simulink model "mpc_model_with_pos_est"  (R2019a)
settings: Solver=FixedStepAuto  StartTime=0.0  StopTime=Tfinal  RelTol=1e-3
values from neighbouring files (symbols this model uses):
  A = [-0.0285 -0.0014; -0.0371 -0.1476]    [model.m]
  DCLINK_Cap = 1000e-12    (= 1e-09)    [mpc_model_parameters.m]    (also in mpc_model_parameters_dual_module.m = 0.001)
  FaultTime = 50    [mpc_model_parameters.m]
  FluxPM = MeanInducedVoltagePeak/(2*pi*100)    [mpc_model_parameters.m]    (also in mpc_model_parameters_dual_module.m)
  Inertia = 1e-2    (= 0.01)    [mpc_model_parameters.m]    (also in mpc_model_parameters_dual_module.m)
  iqrated = Trated/(1.5*PolePairs*FluxPM)    [mpc_model_parameters.m]    (also in mpc_model_parameters_dual_module.m)
  MeanLq = (1/12)*(Module1Phase_A_Lq+Module1Phase_B_Lq+Module1Phase_C_Lq+     Module2Phase_A_Lq+Module2Phase_B_Lq+Module2Phase_C_Lq+     Module3Phase_A_Lq+Module3Phase_B_Lq+Module3Phase_C_Lq+     Module4Phase_A_Lq+Module4Phase_B_Lq+Module4Phase_C_Lq)    [mpc_model_parameters.m]    (also in mpc_model_parameters_dual_module.m)
  PolePairs = 10    [mpc_model_parameters.m]    (also in mpc_model_parameters_dual_module.m)
  Rin = 1e-3    (= 0.001)    [mpc_model_parameters.m]    (also in mpc_model_parameters_dual_module.m)
  Rs = 0.531    [Loss_Distribution.m]    (also in MPC_id_iq.m; mpc_model_parameters.m = 0.321; mpc_model_parameters_dual_module.m = 0.539)
  Sampling_time = 1e-6    (= 1e-06)    [mpc_model_parameters.m]    (also in mpc_model_parameters_dual_module.m)
  SpeedRef1 = 50    [mpc_model_parameters.m]    (also in mpc_model_parameters_dual_module.m = 35)
  SpeedRef2 = 100    [mpc_model_parameters.m]    (also in mpc_model_parameters_dual_module.m = 35)
  SpeedRefUpdateTime = 0.25    [mpc_model_parameters.m]    (also in mpc_model_parameters_dual_module.m = 1.75)
  Tload1 = 5    [mpc_model_parameters.m]    (also in mpc_model_parameters_dual_module.m = 30)
  Tload2 = 10    [mpc_model_parameters.m]    (also in mpc_model_parameters_dual_module.m = 63.6619772368)
  TloadUpdateTime = 0.5    [mpc_model_parameters.m]    (also in mpc_model_parameters_dual_module.m)
  Vdc = 50    [mpc_model_parameters.m]    (also in mpc_model_parameters_dual_module.m = 40)
  Vin = Vdc + Rin*(Pout/Vdc)    (= 50.04)    [mpc_model_parameters.m]    (also in mpc_model_parameters_dual_module.m = 40.05)
  ViscousFriction = 1e-3    (= 0.001)    [mpc_model_parameters.m]    (also in mpc_model_parameters_dual_module.m)
undefined symbols (not defined in the file or in its folder): DiscIntNeverNeededParam
libraries: powerlib x16, dspswit3 x6, simulink x2, powerlib_meascontrol x2
settings Model: Creator=hakan  LastModifiedBy=hakan
settings SolverCC: ZeroCrossAlgorithm=Adaptive
settings DebuggingCC: IgnoredZcDiagnostic=none

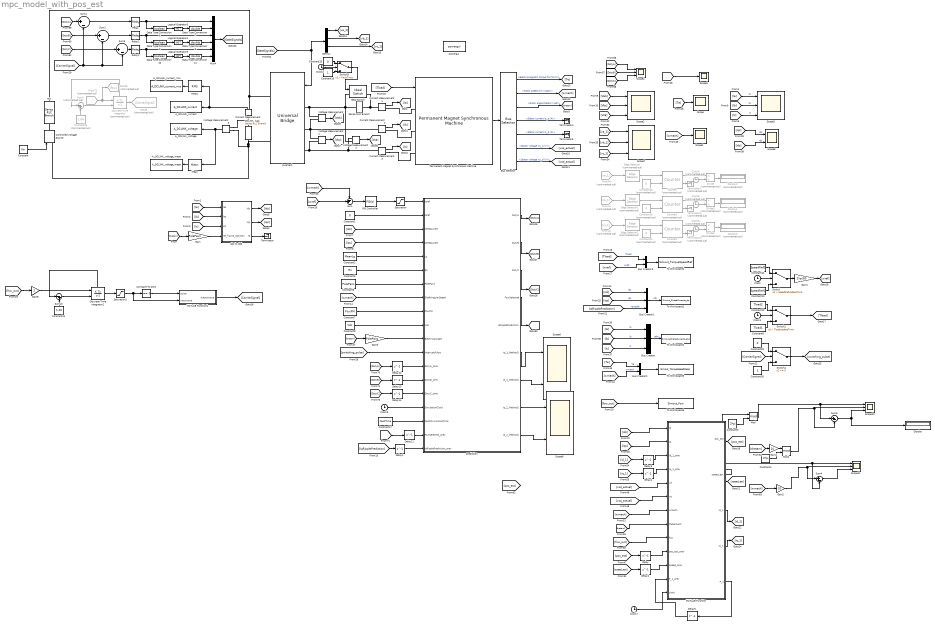
== system mpc_model_with_pos_est ==
  A_DCLINK_current : ToWorkspace  VariableName=A_DCLINK_current  SaveFormat=Structure With Time  SampleTime=-1
  A_DCLINK_current_rms : ToWorkspace  VariableName=A_DCLINK_current_rms  SaveFormat=Structure With Time  SampleTime=-1
  A_DCLINK_voltage : ToWorkspace  VariableName=A_DCLINK_voltage  SaveFormat=Structure With Time  SampleTime=-1
  A_DCLINK_voltage_mean : ToWorkspace  VariableName=A_DCLINK_voltage_mean  SaveFormat=Structure With Time  SampleTime=-1
  Bus Creator : BusCreator  Inputs=3
  Bus Creator1 : BusCreator  Inputs=3
  Bus Creator2 : BusCreator  Inputs=2
  Bus Creator3 : BusCreator  Inputs=2
  Bus Selector : BusSelector  OutputSignals=Electromagnetic torque Te (N*m),Rotor speed wm (rad/s),Rotor angle thetam (rad),Stator current is_q (A),Stator current is_d (A),Stator voltage Vs_q (V),Stator voltage Vs_d (V)
  Clock{,1..3,7} (5 alike) : Clock
  Clock4 : Clock  Commented=on
  Clock5 : Clock  Commented=on
  Clock6 : Clock  Commented=on
  Compare To Zero : simulink/Logic and Bit Operations/Compare To Zero  relop===  OutDataTypeStr=boolean
  Constant : Constant  Value=Vin
  Constant1 : Constant  Value=0
  Constant10 : Constant  Value=SpeedRef1
  Constant11 : Constant  Value=SpeedRef2
  Constant12 : Constant  Value=Tload2
  Constant15 : Constant  Value=0
  Constant16 : Constant
  Constant17 : Constant  Value=FaultTime
  Constant18 : Constant  Commented=on  Value=0
  Constant19 : Constant  Commented=on  Value=0
  Constant2 : Constant  Value=MeanLq
  Constant20 : Constant  Commented=on  Value=0
  Constant24 : Constant  Value=1.02
  Constant26 : Constant  Commented=on  Value=1.04
  Constant29 : Constant  Value=0
  Constant3 : Constant  Value=2*pi
  Constant30 : Constant
  Constant4 : Constant  Value=2*pi
  Constant5 : Constant  Value=Rs
  Constant6 : Constant  Value=PolePairs
  Constant7 : Constant  Value=FluxPM
  Constant8 : Constant  Value=Tload1
  Constant9 : Constant  Value=Vdc
  Controlled Voltage Source : powerlib/Electrical Sources/Controlled Voltage Source  Initialize=on  Source_Type=DC  Amplitude=Vin  Phase=0  Frequency=0  Measurements=None
      settings: SourceProductName=Simscape Electrical
  Counter : dspswit3/Counter  Commented=on  Direction=Up  CountEvent=Rising edge  CounterSize=User defined  MaxCount=9999999999999999999  InitialCount=0  Output=Count and Hit  HitValue=32  ResetInput=on  SamplesPerFrame=1  Ts=1  CntDtype=double  HitDtype=Logical
  Counter1 : dspswit3/Counter  Commented=on  Direction=Up  CountEvent=Rising edge  CounterSize=User defined  MaxCount=9999999999999999999  InitialCount=0  Output=Count and Hit  HitValue=32  ResetInput=on  SamplesPerFrame=1  Ts=1  CntDtype=double  HitDtype=Logical
  Counter2 : dspswit3/Counter  Commented=on  Direction=Up  CountEvent=Rising edge  CounterSize=User defined  MaxCount=9999999999999999999  InitialCount=0  Output=Count and Hit  HitValue=32  ResetInput=on  SamplesPerFrame=1  Ts=1  CntDtype=double  HitDtype=Logical
  Current Measurement{,1..3} (4 alike) : powerlib/Measurements/Current Measurement  PhasorSimulation=off  OutputType=Complex  PSBequivalent=0
      settings: SourceProductName=Simscape Electrical
  DCLINK_Cap : powerlib/Elements/Series RLC Branch  LConnTagsString=__new0  RConnTagsString=__new0  BranchType=C  Resistance=1  Inductance=1e-3  SetiL0=off  InitialCurrent=0  Capacitance=DCLINK_Cap  Setx0=on  InitialVoltage=Vin  Measurements=None
      settings: SourceProductName=Simscape Electrical
  Data Type Conversion10 : DataTypeConversion  OutDataTypeStr=boolean
  Data Type Conversion11 : DataTypeConversion  OutDataTypeStr=double
  Data Type Conversion6 : DataTypeConversion  OutDataTypeStr=boolean
  Data Type Conversion7 : DataTypeConversion  OutDataTypeStr=double
  Data Type Conversion8 : DataTypeConversion  OutDataTypeStr=boolean
  Data Type Conversion9 : DataTypeConversion  OutDataTypeStr=double
  Delay{,1..5,11..14} (10 alike) : Delay  DelayLength=1
  Demux : Demux  Outputs=6
  Discrete-Time Integrator : DiscreteIntegrator  Commented=on  ExternalReset=falling  SampleTime=-1  ShowStatePort=on  ICPrevOutput=DiscIntNeverNeededParam  ICPrevScaledInput=DiscIntNeverNeededParam
  Discrete-Time Integrator2 : DiscreteIntegrator  ExternalReset=falling  SampleTime=Sampling_time  UpperSaturationLimit=1  LowerSaturationLimit=0  ShowStatePort=on  ICPrevOutput=DiscIntNeverNeededParam  ICPrevScaledInput=DiscIntNeverNeededParam
  Display : Display
  Display1 : Display  Commented=on
  Display2 : Display  Commented=on
  Display3 : Display  Commented=on
  Divide : Product  Commented=on  Inputs=*/
  Divide1 : Product  Commented=on  Inputs=*/
  Divide2 : Product  Commented=on  Inputs=*/
  Edge Detector : dspswit3/Edge Detector  Commented=on  InputProcessing=Columns as channels (frame based)
      settings: SourceProductName=DSP System Toolbox  SourceProductBaseCode=DS
  Edge Detector1 : dspswit3/Edge Detector  Commented=on  InputProcessing=Columns as channels (frame based)
      settings: SourceProductName=DSP System Toolbox  SourceProductBaseCode=DS
  Edge Detector2 : dspswit3/Edge Detector  Commented=on  InputProcessing=Columns as channels (frame based)
      settings: SourceProductName=DSP System Toolbox  SourceProductBaseCode=DS
  From40 : From  Commented=on  GotoTag=va_1
  From41 : From  Commented=on  GotoTag=vb_1
  From42 : From  Commented=on  GotoTag=vc_1
  From72 : From  Commented=on  GotoTag=fsw_out
  Gain : Gain  Gain=PolePairs
  Gain1 : Gain  Gain=2*pi/60
  Gain2 : Gain  Gain=10
  Gain3 : Gain  Gain=PolePairs
  Gain4 : Gain  Gain=10
  Gain8 : Gain  Gain=2
  Goto29 : Goto  Commented=on  GotoTag=fsw
  Goto9 : Goto  Commented=on  GotoTag=CarrierSignal
  Ideal Switch : powerlib/Power Electronics/Ideal Switch  Ron=0.001  Lon=0  IC=0  Rs=1e5  Cs=inf  Measurements=on
      settings: SourceProductName=Simscape Electrical
  Inverter1 : powerlib/Power Electronics/Universal Bridge  Arms=3  SnubberResistance=1e5  SnubberCapacitance=inf  Device=IGBT / Diodes  Ron=0.65e-3  Lon=0  ForwardVoltages="[  0  0  ]"  ForwardVoltage=0  GTOparameters=[ 10e-6 , 20e-6 ]  IGBTparameters=[ 1e-6 , 2e-6 ]  Measurements=All voltages and currents  Measurements_2=None  converterType=Rectifier
      settings: SourceProductName=Simscape Electrical
  Logical Operator3 : Logic  Operator=NOT  AllPortsSameDT=off  OutDataTypeStr=boolean
  Logical Operator4 : Logic  Operator=NOT  AllPortsSameDT=off  OutDataTypeStr=boolean
  Logical Operator5 : Logic  Operator=NOT  AllPortsSameDT=off  OutDataTypeStr=boolean
  MATLAB Function : MATLAB Function  TreatAsAtomicUnit=on
  MATLAB Function1 : MATLAB Function  TreatAsAtomicUnit=on
  Mean : powerlib_meascontrol/Measurements/Mean  Freq=THD_mean_frequency  Vinit=0  Ts=0
      settings: SourceProductName=Simscape Electrical
  Mod : Math  Operator=mod  SaturateOnIntegerOverflow=on
  Mod1 : Math  Operator=mod  SaturateOnIntegerOverflow=on
  Mux4 : Mux  Inputs=6
  PID Controller : simulink/Continuous/PID Controller  Controller=PID  Form=Parallel  TimeDomain=Continuous-time  SampleTime=-1  IntegratorMethod=Forward Euler  FilterMethod=Forward Euler  ControllerParametersSource=internal  P=1  I=10  D=0  UseFilter=on  N=100  TunerSelectOption=Transfer Function Based (PID Tuner App)  InitialConditionSource=internal  InitialConditionForIntegrator=0  InitialConditionForFilter=0  DifferentiatorICPrevScaledInput=0  ExternalReset=none  TrackingMode=off  Kt=1  LimitOutput=off  UpperSaturationLimit=inf  LowerSaturationLimit=-inf  LinearizeAsGain=on  AntiWindupMode=none  Kb=1  POutMin=[]  POutMax=[]  IOutMin=[]  IOutMax=[]  DOutMin=[]  DOutMax=[]  NOutMin=[]  NOutMax=[]  SumOutMin=[]  SumOutMax=[]  SaturationOutMin=[]  SaturationOutMax=[]  PParamMin=[]  PParamMax=[]  IParamMin=[]  IParamMax=[]  DParamMin=[]  DParamMax=[]  NParamMin=[]  NParamMax=[]  KbParamMin=[]  KbParamMax=[]  KtParamMin=[]  KtParamMax=[]  KbOutMin=[]  KbOutMax=[]  KtOutMin=[]  KtOutMax=[]  IntegratorOutMin=[]  IntegratorOutMax=[]  FilterOutMin=[]  FilterOutMax=[]  SumI1OutMin=[]  SumI1OutMax=[]  SumI2OutMin=[]  SumI2OutMax=[]  SumI3OutMin=[]  SumI3OutMax=[]  SumI4OutMin=[]  SumI4OutMax=[]  SumDOutMin=[]  SumDOutMax=[]  DifferentiatorOutMin=[]  DifferentiatorOutMax=[]  FilterDiffOutCoefMin=[]  FilterDiffOutCoefMax=[]  ReciprocalOutMin=[]  ReciprocalOutMax=[]  SumDenOutMin=[]  SumDenOutMax=[]  SumNumOutMin=[]  SumNumOutMax=[]  DivideOutMin=[]  DivideOutMax=[]  IntegratorContinuousStateAttributes=''  IntegratorStateMustResolveToSignalObject=off  IntegratorRTWStateStorageClass=Auto  FilterContinuousStateAttributes=''  FilterStateMustResolveToSignalObject=off  FilterRTWStateStorageClass=Auto  ParallelPVariant=InternalParameters  IdealPVariant=Disabled  IVariant=InternalParameters  DVariant=InternalParameters  IntegratorVariant=Continuous  SatVariant=Disabled  AWVariant=Passthrough  PCopyVariant=Disabled  TRVariant=Disabled  FdbkBlocksVariant=Forward  IdealPFdbkVariant=Disabled  SatFdbkVariant=Disabled  DerivativeFilterVariant=ContFilter  NVariant=InternalParameters  NCopyVariant=Disabled  FilterICVariant=InternalICsFilter  IntegratorICVariant=InternalICs  ExternalResetVariant=Disabled  TRSumVariant=Passthrough  SumFdbkVariant=Disabled  SumVariant=Sum_PID
  Permanent Magnet Synchronous Machine : powerlib/Machines/Permanent Magnet Synchronous Machine  NbPhases=3  FluxDistribution=Sinusoidal  RotorType=Round  MechanicalLoad=Torque Tm  PresetModel=No  ShowDetailedParameters=on  MeasurementBus=off  Resistance=Rs  Inductance=8.5e-3  dqInductances=[3.1e-3,3.6e-3]  La=Ls  MachineConstant=Voltage Constant (V_peak L-L / krpm)  Flux=0.18074  VoltageCst=VoltageConstant  TorqueCst=2.7111  Flat=120  Mechanical=[Inertia ViscousFriction PolePairs 0]  PolePairs=4  InitialConditions=[0*100*2*pi/60,0, 0,0]  InitialConditions5ph=[0 0 0 0 0 0]  TsPowergui=0  TsBlock=-1  RefAngle=90 degrees behind phase A axis (modified Park)
  RMS1 : powerlib_meascontrol/Measurements/RMS  TrueRMS=on  Freq=Load_Nominal_Freq  RMSInit=10  Ts=0
      settings: SourceProductName=Simscape Electrical
  Relay : Relay
  Relay1 : Relay
  Relay2 : Relay
  Rin : powerlib/Elements/Series RLC Branch  LConnTagsString=__new0  RConnTagsString=__new0  BranchType=R  Resistance=Rin  Inductance=1e-3  SetiL0=off  InitialCurrent=0  Capacitance=1000e-6  Setx0=off  InitialVoltage=0  Measurements=None
      settings: SourceProductName=Simscape Electrical
  Saturation : Saturate  UpperLimit=2*iqrated  LowerLimit=-2*iqrated  LinearizeAsGain=off
  Saturation1 : Saturate  UpperLimit=1  LowerLimit=0
  Scope : Scope
  Scope1 : Scope
  Scope{2..4,7,10..11} (6 alike) : Scope  NumInputPorts=3
  Scope5 : Scope
  Scope6 : Scope  NumInputPorts=2
  Scope8 : Scope  NumInputPorts=2
  Scope9 : Scope  NumInputPorts=2
  Series RLC Branch : powerlib/Elements/Series RLC Branch  LConnTagsString=__new0  RConnTagsString=__new0  BranchType=R  Resistance=5000  Inductance=1e-3  SetiL0=off  InitialCurrent=0  Capacitance=1e-6  Setx0=off  InitialVoltage=0  Measurements=None
      settings: SourceProductName=Simscape Electrical
  Sum : Sum  Inputs=-+|
  Sum{1..2,4..6} (5 alike) : Sum  Inputs=|+-
  Sum10 : Sum  Inputs=|-+
  Sum3 : Sum  Commented=on  Inputs=|-+
  Switch : Switch  Criteria=u2 > Threshold  Threshold=SpeedRefUpdateTime
  Switch1 : Switch  Criteria=u2 > Threshold  Threshold=TloadUpdateTime
  Switch3 : Switch  Criteria=u2 > Threshold  Threshold=FaultTime
  Switch4 : Switch  Criteria=u2 ~= 0
  Terminator : Terminator
  Terminator1 : Terminator  Commented=on
  Terminator2 : Terminator  Commented=on
  Terminator3 : Terminator  Commented=on
  Terminator4 : Terminator
  Terminator5 : Terminator
  To Workspace1 : ToWorkspace  VariableName=Simout_PhaseCurrents_abc  SaveFormat=Timeseries  SampleTime=-1
  To Workspace2 : ToWorkspace  VariableName=Simout_PhaseCurrents_dq  SaveFormat=Timeseries  SampleTime=-1
  To Workspace3 : ToWorkspace  VariableName=Simout_TorqueSpeedMeas  SaveFormat=Timeseries  SampleTime=-1
  To Workspace4 : ToWorkspace  VariableName=Simout_TorqueSpeedRef  SaveFormat=Timeseries  SampleTime=-1
  To Workspace5 : ToWorkspace  VariableName=Simout_Fsw  SaveFormat=Timeseries  SampleTime=-1
  Voltage Measurement{,1..3} (4 alike) : powerlib/Measurements/Voltage Measurement  PhasorSimulation=off  OutputType=Complex  PSBequivalent=0
      settings: SourceProductName=Simscape Electrical
  abc to dq0 : MATLAB Function  TreatAsAtomicUnit=on
  powergui : powerlib/powergui  Priority=1  SimulationMode=Discrete  SampleTime=Sampling_time  frequency=60  Iterations=50  frequencyindice=0  Pbase=100e6  ErrMax=1e-4  UnitsV=kV  UnitsW=MW  buscounter=0  FunctionMessages=off  echomessages=off  EnableUseOfTLC=off  CurrentSourceSwitches=off  DisableSnubberDevices=off  DisableRonSwitches=off  DisableVfSwitches=off  DisplayEquations=off  AutomaticDiscreteSolvers=off  SolverType=Tustin/Backward Euler (TBE)  Interpol=off  ExternalGateDelay=off  methode=off  Ts=100  x0status=blocks  SPID=on  SwTol=0  HookPort=off  NonlinearTolerance=0  nMaxIteration=15  ContinueOnMaxIteration=off  RestoreLinks=warning  ResistiveCurrentMeasurement=off  Frange=[0:2:500]  Ylog=off  Xlog=on  ShowGrid=off  save=off  variable=ZData  structure=0  ZoomFFT=off  StartTime=0.0  cycles=1  DisplayStyle=1  fundamental=60  FreqAxis=off  MaxFrequency=1000  frequencyindicesteady=1  RmsSteady=1  display=off
      settings: SourceProductName=Simscape Electrical
  prediction : MATLAB Function  TreatAsAtomicUnit=on
  wires:
  Voltage Measurement3/1 -> Mean/1, A_DCLINK_voltage/1
  RMS1/1 -> A_DCLINK_current_rms/1
  Constant/1 -> Controlled Voltage Source/1
  Mean/1 -> A_DCLINK_voltage_mean/1
  Current Measurement/1 -> RMS1/1, A_DCLINK_current/1
  Permanent Magnet Synchronous Machine/1 -> Bus Selector/1
  Bus Selector/1 -> [Te]  "<Electromagnetic torque Te (N*m)>"
  Bus Selector/2 -> [wmech]  "<Rotor speed wm (rad/s)>"
  Current Measurement1/1 -> [Ia]
  Current Measurement2/1 -> [Ib]
  Current Measurement3/1 -> [Ic]
  Bus Selector/3 -> [thetam]  "<Rotor angle thetam (rad)>"
  [thetam] -> Gain/1
  [Ia] -> abc to dq0/1(ias)
  [Ib] -> abc to dq0/2(ibs)
  [Ic] -> abc to dq0/3(ics)
  Gain/1 -> abc to dq0/4(ref_frame_position)
  Bus Selector/4 -> Terminator4/1  "<Stator current is_q (A)>"
  Bus Selector/5 -> Terminator5/1  "<Stator current is_d (A)>"
  abc to dq0/2(iqs) -> [iqs]
  abc to dq0/1(ids) -> [ids]
  abc to dq0/3(i0) -> Terminator/1
  [ids] -> prediction/3(IdMeasured)
  [iqs] -> prediction/4(IqMeasured)
  Constant2/1 -> prediction/5(Ls)
  Voltage Measurement/1 -> [Vab]
  Voltage Measurement1/1 -> [Vbc]
  Voltage Measurement2/1 -> [Vca]
  Bus Selector/6 -> [vsq_actual]  "<Stator voltage Vs_q (V)>"
  Bus Selector/7 -> [vsd_actual]  "<Stator voltage Vs_d (V)>"
  [Vca] -> Scope2/3
  [Vbc] -> Scope2/2
  [Vab] -> Scope2/1
  Constant5/1 -> prediction/6(Rs)
  Constant6/1 -> prediction/7(PolePairs)
  [wmech] -> prediction/8(ShaftAngularSpeed)
  Constant7/1 -> prediction/9(FluxPM)
  Constant9/1 -> prediction/10(Vdc)
  Gain3/1 -> prediction/11(ElectricalAngle)
  [thetam] -> Gain3/1
  [Tload] -> Permanent Magnet Synchronous Machine/1
  PID Controller/1 -> Saturation/1
  Sum/1 -> PID Controller/1
  [wmech] -> Sum/1
  [iqs] -> Bus Creator1/2  "iqs"
  [ids] -> Bus Creator1/1  "ids"
  Constant10/1 -> Switch/3
  Constant11/1 -> Switch/1
  Switch/1 -> Gain1/1
  Clock/1 -> Switch/2
  Clock1/1 -> Switch1/2
  Constant12/1 -> Switch1/1
  Constant8/1 -> Switch1/3
  Switch1/1 -> [Tload]
  Bus Creator/1 -> To Workspace1/1  "Iabc"
  Bus Creator1/1 -> To Workspace2/1  "Idq"
  Bus Creator2/1 -> To Workspace3/1
  [wref] -> Sum/2
  Gain1/1 -> [wref]
  [Tload] -> Bus Creator3/1  "Tload"
  [wref] -> Bus Creator3/2  "wref"
  Bus Creator3/1 -> To Workspace4/1
  [switching_pulse] -> prediction/12(InterruptPulse)
  Clock2/1 -> Switch3/2
  Constant15/1 -> Switch3/1
  Constant16/1 -> Switch3/3
  Switch3/1 -> Ideal Switch/1
  Clock3/1 -> prediction/16(SimulationClock)
  Constant17/1 -> prediction/17(FaultOccuranceTime)
  [va_1] -> Scope7/1
  [vb_1] -> Scope7/2
  [vc_1] -> Scope7/3
  Edge Detector/1 -> Counter/1
  Constant18/1 -> Counter/2
  Counter/1 -> Divide/1
  Clock4/1 -> Divide/2
  Divide/1 -> Display2/1
  [Ib] -> Bus Creator/2  "Ib"
  [Ia] -> Bus Creator/1  "Ia"
  [Ic] -> Bus Creator/3  "Ic"
  [Ib] -> Scope3/2  "Ib"
  [Ic] -> Scope3/3  "Ic"
  [Ia] -> Scope3/1  "Ia"
  [iqs] -> Scope8/1  "iqs"
  [ids] -> Scope8/2  "ids"
  Counter/2 -> Terminator1/1
  From40/1 -> Edge Detector/1
  From41/1 -> Edge Detector1/1
  Counter1/2 -> Terminator2/1
  Divide1/1 -> Display1/1
  Clock5/1 -> Divide1/2
  Counter1/1 -> Divide1/1
  Constant19/1 -> Counter1/2
  Edge Detector1/1 -> Counter1/1
  Edge Detector2/1 -> Counter2/1
  Constant20/1 -> Counter2/2
  Counter2/1 -> Divide2/1
  Clock6/1 -> Divide2/2
  Divide2/1 -> Display3/1
  Counter2/2 -> Terminator3/1
  From42/1 -> Edge Detector2/1
  [Te] -> Bus Creator2/1  "Te"
  [wmech] -> Bus Creator2/2  "wmech"
  [Te] -> Scope/1
  [wmech] -> Scope1/1
  prediction/1(DutyA) -> [DutyA]
  prediction/3(DutyC) -> [DutyC]
  prediction/2(DutyB) -> [DutyB]
  [DutyB] -> Scope4/2
  [DutyA] -> Scope4/1
  [DutyC] -> Scope4/3
  Constant26/1 -> Sum3/2
  From72/1 -> Goto29/1, Discrete-Time Integrator/1
  Discrete-Time Integrator/State -> Sum3/1
  Sum3/1 -> Discrete-Time Integrator/2
  Switch4/1 -> [switching_pulse]
  Constant30/1 -> Switch4/3
  Constant29/1 -> Switch4/1
  [GateSignals] -> Inverter1/1, Demux/1
  Demux/1 -> [va_1]
  Demux/3 -> [vb_1]
  prediction/4(FswSelected) -> [fsw_out]
  Delay11/1 -> prediction/18(FswSelected_prev)
  [fsw_out] -> Delay11/1
  [DutyB] -> Delay13/1
  [DutyA] -> Delay12/1
  [DutyC] -> Delay14/1
  Delay13/1 -> prediction/14(DutyB_prev)
  Delay12/1 -> prediction/13(DutyA_prev)
  Delay14/1 -> prediction/15(DutyC_prev)
  Discrete-Time Integrator/1 -> Goto9/1
  [CarrierSignal] -> Switch4/2
  Demux/5 -> [vc_1]
  [IqRipplePrediction] -> Delay1/1
  Delay1/1 -> prediction/19(IqRipplePrediction_prev)
  [CarrierSignal] -> Sum1/2, Sum2/2, Sum5/2
  Logical Operator4/1 -> Data Type Conversion9/1
  [DutyA] -> Sum1/1
  Data Type Conversion8/1 -> Logical Operator4/1
  Data Type Conversion10/1 -> Logical Operator5/1
  Relay1/1 -> Data Type Conversion8/1, Mux4/3
  Relay2/1 -> Data Type Conversion10/1, Mux4/5
  Data Type Conversion6/1 -> Logical Operator3/1
  Sum1/1 -> Relay/1
  Data Type Conversion11/1 -> Mux4/6
  [DutyC] -> Sum5/1
  Relay/1 -> Mux4/1, Data Type Conversion6/1
  Data Type Conversion9/1 -> Mux4/4
  Sum5/1 -> Relay2/1
  Logical Operator3/1 -> Data Type Conversion7/1
  Logical Operator5/1 -> Data Type Conversion11/1
  Sum2/1 -> Relay1/1
  Mux4/1 -> [GateSignals]
  [DutyB] -> Sum2/1
  Data Type Conversion7/1 -> Mux4/2
  [fsw_out] -> Scope5/1
  Saturation/1 -> prediction/1(iqref)
  Discrete-Time Integrator2/State -> Sum10/1
  Gain8/1 -> Discrete-Time Integrator2/1
  Sum10/1 -> Discrete-Time Integrator2/2
  [fsw_out] -> Gain8/1
  Saturation1/1 -> MATLAB Function1/2(inputwave), Compare To Zero/1
  Constant24/1 -> Sum10/2
  Discrete-Time Integrator2/1 -> Saturation1/1
  Compare To Zero/1 -> MATLAB Function1/1(pulse)
  MATLAB Function1/1(outputwave) -> [CarrierSignal]
  [fsw_out] -> To Workspace5/1
  [IqRipplePrediction] -> Bus Creator1/3  "iqripple"
  Constant1/1 -> prediction/2(idref)
  prediction/7(Id_1_Method1) -> Scope6/2
  prediction/6(Iq_1_Method1) -> Scope6/1
  prediction/8(Iq_2_Method1) -> Scope9/1
  prediction/9(Id_2_Method1) -> Scope9/2
  [ids] -> MATLAB Function/1(id)
  [iqs] -> MATLAB Function/2(iq)
  MATLAB Function/1(pos_est) -> [pos_est], Mod/1
  Delay/1 -> MATLAB Function/10(pos_est_prev)
  [pos_est] -> Delay/1
  Delay2/1 -> MATLAB Function/11(speed_prev)
  [speed_est] -> Delay2/1
  [vsq_actual] -> MATLAB Function/6(vq)
  [vsd_actual] -> MATLAB Function/5(vd)
  [fsw_out] -> MATLAB Function/9(fsw)
  [wmech] -> MATLAB Function/7(wmech)
  [thetam] -> MATLAB Function/8(thetamech)
  MATLAB Function/3(id_1) -> [id_1]
  MATLAB Function/4(iq_1) -> [iq_1]
  Delay3/1 -> MATLAB Function/3(id_1_prev)
  [id_1] -> Delay3/1
  [iq_1] -> Delay4/1
  Delay4/1 -> MATLAB Function/4(iq_1_prev)
  Mod/1 -> Sum6/1, Scope10/1
  Constant3/1 -> Mod/2
  MATLAB Function/2(speed_est) -> [speed_est], Sum4/2, Scope11/1
  [wmech] -> Gain2/1
  Gain2/1 -> Sum4/1, Scope11/2
  Constant4/1 -> Mod1/2
  Mod1/1 -> Sum6/2, Scope10/2
  [thetam] -> Gain4/1
  Gain4/1 -> Mod1/1
  MATLAB Function/5(P_1) -> Delay5/1
  Delay5/1 -> MATLAB Function/12(P_1_prev)
  Clock7/1 -> MATLAB Function/13(clock)
  Sum4/1 -> Scope11/3
  Sum6/1 -> Display/1, Scope10/3
  connections:
  Rin/LConn1 -- Current Measurement/RConn1 -- Inverter1/RConn1
  Controlled Voltage Source/LConn1 -- Voltage Measurement3/LConn2 -- DCLINK_Cap/RConn1 -- Inverter1/RConn2
  DCLINK_Cap/LConn1 -- Current Measurement/LConn1 -- Voltage Measurement3/LConn1
  Controlled Voltage Source/RConn1 -- Rin/RConn1
  Voltage Measurement2/LConn2 -- Ideal Switch/LConn1 -- Series RLC Branch/LConn1 -- Voltage Measurement/LConn1 -- Inverter1/LConn1
  Current Measurement2/LConn1 -- Voltage Measurement1/LConn1 -- Voltage Measurement/LConn2 -- Inverter1/LConn2
  Inverter1/LConn3 -- Voltage Measurement1/LConn2 -- Voltage Measurement2/LConn1 -- Current Measurement3/LConn1
  Current Measurement3/RConn1 -- Permanent Magnet Synchronous Machine/LConn3
  Permanent Magnet Synchronous Machine/LConn2 -- Current Measurement2/RConn1
  Permanent Magnet Synchronous Machine/LConn1 -- Current Measurement1/RConn1
  Current Measurement1/LConn1 -- Ideal Switch/RConn1 -- Series RLC Branch/RConn1

== matlab function mpc_model_with_pos_est/prediction ==
  data: DutyA output; DutyB output; DutyC output; iqref input; idref input; IdMeasured input; IqMeasured input; Ls input; Rs input; PolePairs input; ShaftAngularSpeed input; FluxPM input; Vdc input; ElectricalAngle input; InterruptPulse input; DutyA_prev input; DutyB_prev input; DutyC_prev input; SimulationClock input; FaultOccuranceTime input; FswSelected_prev input; FswSelected output; IqRipplePrediction output; IqRipplePrediction_prev input; Iq_1_Method1 output; Id_1_Method1 output; Iq_2_Method1 output; Id_2_Method1 output
function [DutyA, DutyB, DutyC, FswSelected, IqRipplePrediction,Iq_1_Method1,Id_1_Method1,Iq_2_Method1,Id_2_Method1]  = fcn(iqref,idref,IdMeasured, IqMeasured, Ls, Rs,PolePairs,ShaftAngularSpeed,FluxPM,Vdc,ElectricalAngle,InterruptPulse,DutyA_prev, DutyB_prev, DutyC_prev, SimulationClock,FaultOccuranceTime,FswSelected_prev, IqRipplePrediction_prev)
Ld = Ls;
Lq = Ls;
I_Normalize = 11.7362; %this is the rated value of the IqMeasured
cost = zeros(1,8);
VdPrediction_1 = zeros(1,8);
VqPrediction_1 = zeros(1,8);
% FswOptions = [5000; 10000; 15000; 20000; 25000; 30000; 35000; 40000];
FswMax = 40000;
FswOptions = 1000:1000:FswMax;
cost = zeros(1,numel(FswOptions));
VdPrediction_1 = zeros(1,numel(FswOptions));
VqPrediction_1 = zeros(1,numel(FswOptions));
VdPrediction_2 = zeros(1,numel(FswOptions));
VqPrediction_2 = zeros(1,numel(FswOptions));
IqRipplePredictionArray_1 = zeros(1,numel(FswOptions));
IqRipplePredictionArray_2 = zeros(1,numel(FswOptions));
VoltageDuring_T1_1 = zeros(1,numel(FswOptions));
VoltageDuring_T2_1 = zeros(1,numel(FswOptions));
VoltageDuring_T0_1 = zeros(1,numel(FswOptions));
VoltageDuring_T1_2 = zeros(1,numel(FswOptions));
VoltageDuring_T2_2 = zeros(1,numel(FswOptions));
VoltageDuring_T0_2 = zeros(1,numel(FswOptions));
MagnitudePrediction_1 = zeros(1,numel(FswOptions));
MagnitudePrediction_2 = zeros(1,numel(FswOptions));

SvpwmT1Prediction_1 =  zeros(1,numel(FswOptions));
SvpwmT2Prediction_1 =  zeros(1,numel(FswOptions));
SvpwmT0Prediction_1 =  zeros(1,numel(FswOptions));

SvpwmT1Prediction_2 =  zeros(1,numel(FswOptions));
SvpwmT2Prediction_2 =  zeros(1,numel(FswOptions));
SvpwmT0Prediction_2 =  zeros(1,numel(FswOptions));

ValfaPrediction_1 = zeros(1,numel(FswOptions)); 
VbetaPrediction_1 = zeros(1,numel(FswOptions)); 
ValfaPrediction_2 = zeros(1,numel(FswOptions)); 
VbetaPrediction_2 = zeros(1,numel(FswOptions)); 
maPrediction_1 = zeros(1,numel(FswOptions)); 
maPrediction_2 = zeros(1,numel(FswOptions));

IqDelta_Prediction_During_T1_1 =  zeros(1,numel(FswOptions));
IqDelta_Prediction_During_T2_1 =  zeros(1,numel(FswOptions));
IqDelta_Prediction_During_T0_1 =  zeros(1,numel(FswOptions));
IqDelta_Prediction_During_T1_2 =  zeros(1,numel(FswOptions));
IqDelta_Prediction_During_T2_2 =  zeros(1,numel(FswOptions));
IqDelta_Prediction_During_T0_2 =  zeros(1,numel(FswOptions));
VoltageVectorAnglePredictionMod_1 = zeros(1,numel(FswOptions));
VoltageVectorAnglePrediction_1 = zeros(1,numel(FswOptions));
VoltageVectorAnglePredictionMod_2 = zeros(1,numel(FswOptions));
VoltageVectorAnglePrediction_2 = zeros(1,numel(FswOptions));

IdPrediction_1_array = zeros(1,numel(FswOptions));
IqPrediction_1_array = zeros(1,numel(FswOptions));
IdPrediction_2_array = zeros(1,numel(FswOptions));
IqPrediction_2_array = zeros(1,numel(FswOptions));

IqRippleCoeff = 10000;
IqRefCoeff = 100000;
IdRefCoeff = 15;
FswCoeff = 1500;
Iq_1_Method1 = 0;
Id_1_Method1 = 0;
Iq_2_Method1 = 0;
Id_2_Method1 = 0;
if(InterruptPulse==1)
    
    for i = 1:numel(FswOptions)
        %% first prediction
        VdPrediction_1(i) = Rs*IdMeasured + Ld*FswOptions(i)*(idref-IdMeasured)-PolePairs*ShaftAngularSpeed*Lq*IqMeasured;
        VqPrediction_1(i) = Rs*IqMeasured + Lq*FswOptions(i)*(iqref-IqMeasured)+PolePairs*ShaftAngularSpeed*(Ld*IdMeasured+FluxPM);
        
        MagnitudePrediction_1(i) = sqrt(VdPrediction_1(i)^2+VqPrediction_1(i)^2);
        
        ValfaPrediction_1(i) = sin(ElectricalAngle)*VdPrediction_1(i)+cos(ElectricalAngle)*VqPrediction_1(i);
        VbetaPrediction_1(i) =-cos(ElectricalAngle)*VdPrediction_1(i)+sin(ElectricalAngle)*VqPrediction_1(i);     
        
        VoltageVectorAnglePrediction_1(i) = atan2(VbetaPrediction_1(i),ValfaPrediction_1(i))+4*pi;
        VoltageVectorAnglePredictionMod_1(i) = mod(VoltageVectorAnglePrediction_1(i),pi/3);
        
        maPrediction_1(i) = MagnitudePrediction_1(i)/(Vdc/sqrt(3));
        
        SvpwmT1Prediction_1(i) = (1/FswOptions(i))*maPrediction_1(i)*sin(pi/3-VoltageVectorAnglePredictionMod_1(i));
        SvpwmT2Prediction_1(i) = (1/FswOptions(i))*maPrediction_1(i)*sin(VoltageVectorAnglePredictionMod_1(i));
        SvpwmT0Prediction_1(i) = (1/FswOptions(i))-SvpwmT1Prediction_1(i)-SvpwmT2Prediction_1(i);        
        
        VoltageDuring_T1_1(i) = 2/3*Vdc-MagnitudePrediction_1(i);
        VoltageDuring_T2_1(i) = 2/3*Vdc-MagnitudePrediction_1(i);
        VoltageDuring_T0_1(i) = -MagnitudePrediction_1(i);
        
        IqDelta_Prediction_During_T1_1(i) = VoltageDuring_T1_1(i)*SvpwmT1Prediction_1(i)/Ls;
        IqDelta_Prediction_During_T2_1(i) = VoltageDuring_T2_1(i)*SvpwmT2Prediction_1(i)/Ls;
        IqDelta_Prediction_During_T0_1(i) = -VoltageDuring_T0_1(i)*SvpwmT0Prediction_1(i)/Ls;
        
        IqRipplePredictionArray_1(i) = IqDelta_Prediction_During_T1_1(i)+IqDelta_Prediction_During_T2_1(i)+IqDelta_Prediction_During_T0_1(i);
        
        %predict the future output
        IdPrediction_1 = IdMeasured + (1/FswOptions(i))*(VdPrediction_1(i)/Ld-Rs/Ld*IdMeasured+Lq/Ld*PolePairs*ShaftAngularSpeed*IqMeasured);
        IqPrediction_1 = IqMeasured + (1/FswOptions(i))*(VqPrediction_1(i)*Lq-Rs/Lq*IqMeasured-Ld/Lq*PolePairs*ShaftAngularSpeed*IdMeasured-FluxPM*PolePairs*ShaftAngularSpeed/Lq);
        TePrediction_1 = 1.5*PolePairs*(FluxPM*IqPrediction_1+0*(Ld-Lq)*IdPrediction_1*IqPrediction_1); % reluctance torque component is multiplied by 0, since it caused unreasonable torque values.
                
        IdPrediction_1_array(i) = IdPrediction_1;
        IqPrediction_1_array(i) = IqPrediction_1;
        
        %% second prediction
        VdPrediction_2(i) = Rs*IdPrediction_1 + Ld*FswOptions(i)*(idref-IdPrediction_1)-PolePairs*ShaftAngularSpeed*Lq*IqPrediction_1;
        VqPrediction_2(i) = Rs*IqPrediction_1 + Lq*FswOptions(i)*(iqref-IqPrediction_1)+PolePairs*ShaftAngularSpeed*(Ld*IdPrediction_1+FluxPM);        
        
        MagnitudePrediction_2(i) = sqrt(VdPrediction_2(i)^2+VqPrediction_2(i)^2);
        
        ValfaPrediction_2(i) = sin(ElectricalAngle)*VdPrediction_2(i)+cos(ElectricalAngle)*VqPrediction_2(i);
        VbetaPrediction_2(i) =-cos(ElectricalAngle)*VdPrediction_2(i)+sin(ElectricalAngle)*VqPrediction_2(i);      
        
        VoltageVectorAnglePrediction_2(i) = atan2(VbetaPrediction_2(i),ValfaPrediction_2(i))+4*pi;
        VoltageVectorAnglePredictionMod_2(i) = mod(VoltageVectorAnglePrediction_2(i),pi/3);   
        
        maPrediction_2(i) = MagnitudePrediction_2(i)/(Vdc/sqrt(3)); 
        
        SvpwmT1Prediction_2(i) = (1/FswOptions(i))*maPrediction_2(i)*sin(pi/3-VoltageVectorAnglePredictionMod_1(i));
        SvpwmT2Prediction_2(i) = (1/FswOptions(i))*maPrediction_2(i)*sin(VoltageVectorAnglePredictionMod_1(i));
        SvpwmT0Prediction_2(i) = (1/FswOptions(i))-SvpwmT1Prediction_2(i)-SvpwmT2Prediction_1(i); 
        
        VoltageDuring_T1_2(i) = 2/3*Vdc-MagnitudePrediction_2(i);
        VoltageDuring_T2_2(i) = 2/3*Vdc-MagnitudePrediction_2(i);
        VoltageDuring_T0_2(i) = -MagnitudePrediction_2(i);
        
        IqDelta_Prediction_During_T1_2(i) = VoltageDuring_T1_2(i)*SvpwmT1Prediction_2(i)/Ls;
        IqDelta_Prediction_During_T2_2(i) = VoltageDuring_T2_2(i)*SvpwmT2Prediction_2(i)/Ls;
        IqDelta_Prediction_During_T0_2(i) = -VoltageDuring_T0_2(i)*SvpwmT0Prediction_2(i)/Ls;        
        
        IqRipplePredictionArray_2(i) = IqDelta_Prediction_During_T1_2(i)+IqDelta_Prediction_During_T2_2(i)+IqDelta_Prediction_During_T0_2(i);
        
        IdPrediction_2 = IdPrediction_1 + (1/FswOptions(i))*(VdPrediction_2(i)/Ld-Rs/Ld*IdPrediction_1+Lq/Ld*PolePairs*ShaftAngularSpeed*IqPrediction_1);
        IqPrediction_2 = IqPrediction_1 + (1/FswOptions(i))*(VqPrediction_2(i)*Lq-Rs/Lq*IqPrediction_1-Ld/Lq*PolePairs*ShaftAngularSpeed*IdPrediction_1-FluxPM*PolePairs*ShaftAngularSpeed/Lq);                
        
        IdPrediction_2_array(i) = IdPrediction_2;
        IqPrediction_2_array(i) = IqPrediction_2;
        
        %% calculate the cost
        if(abs(IqPrediction_1)>30)||(abs(TePrediction_1)>50)
            ProtectionConstant = inf;
        else
            ProtectionConstant = 0;
        end
%         cost(i) = (IqRipplePredictionArray_1(i)/I_Normalize)^2*IqRippleCoeff+IqRefCoeff*((iqref-IqPrediction_1)/I_Normalize)^2+((idref-IdPrediction_1)/I_Normalize)^2*IdRefCoeff+ProtectionConstant+FswOptions(i)/FswMax*FswCoeff;%+IqRipplePrediction_prev^2*100000000;
        cost(i) = (IqRipplePredictionArray_2(i)/I_Normalize)^2*IqRippleCoeff+IqRefCoeff*((iqref-IqPrediction_2)/I_Normalize)^2+((idref-IdPrediction_2)/I_Normalize)^2*IdRefCoeff+ProtectionConstant+FswOptions(i)/FswMax*FswCoeff;%+IqRipplePrediction_prev^2*100000000;
        
    end
    
    [CostMinVal, MinimumCostIndex] = min(cost);
    
    DutyA = 0;
    DutyB = 0;
    DutyC = 0;
    VdsOptimum_1 = VdPrediction_2(MinimumCostIndex);
    VqsOptimum_1 = VqPrediction_2(MinimumCostIndex);
    FswSelected = FswOptions(MinimumCostIndex);
    
    Iq_1_Method1 = IqPrediction_1_array(MinimumCostIndex);
    Id_1_Method1 = IdPrediction_1_array(MinimumCostIndex);

    Iq_2_Method1 = IqPrediction_2_array(MinimumCostIndex);
    Id_2_Method1 = IdPrediction_2_array(MinimumCostIndex);
    
    VoltageVectorAngleOptimum = VoltageVectorAnglePrediction_1(MinimumCostIndex);
    TswSelected = 1/FswSelected;

    
    Svpwm_T1 = SvpwmT1Prediction_2(MinimumCostIndex);
    Svpwm_T2 = SvpwmT2Prediction_2(MinimumCostIndex);
    Svpwm_T0 = SvpwmT0Prediction_2(MinimumCostIndex);
    
    IqRipplePrediction = IqRipplePredictionArray_2(MinimumCostIndex);
    
    if (mod(VoltageVectorAngleOptimum, 2*pi)<=pi/3)&&(mod(VoltageVectorAngleOptimum, 2*pi)>=0)  % sector 1
        DutyA = (Svpwm_T1+Svpwm_T2+Svpwm_T0/2)/TswSelected;
        DutyB = (Svpwm_T2+Svpwm_T0/2)/TswSelected;
        DutyC = (Svpwm_T0/2)/TswSelected;
%         sectornumber = 1;
        return;
    end
    if (mod(VoltageVectorAngleOptimum, 2*pi)<=2*pi/3)&&(mod(VoltageVectorAngleOptimum, 2*pi)>=pi/3)  % sector 2
        DutyA = (Svpwm_T1+Svpwm_T0/2)/TswSelected;
        DutyB = (Svpwm_T1+Svpwm_T2+Svpwm_T0/2)/TswSelected;
        DutyC = (Svpwm_T0/2)/TswSelected;
%         sectornumber = 2;
        return;
    end
    if (mod(VoltageVectorAngleOptimum, 2*pi)<=pi)&&(mod(VoltageVectorAngleOptimum, 2*pi)>=2*pi/3)  % sector 3
        if(mod(VoltageVectorAngleOptimum, pi)==0)
            DutyA = (Svpwm_T0/2)/TswSelected;
            DutyB = (Svpwm_T1+Svpwm_T0/2)/TswSelected;
            DutyC = (Svpwm_T1+Svpwm_T2+Svpwm_T0/2)/TswSelected;
        else
            DutyA = (Svpwm_T0/2)/TswSelected;
            DutyB = (Svpwm_T1+Svpwm_T2+Svpwm_T0/2)/TswSelected;
            DutyC = (Svpwm_T2+Svpwm_T0/2)/TswSelected;
        end
%         sectornumber = 3;
        return;
    end
    if (mod(VoltageVectorAngleOptimum, 2*pi)<=4*pi/3)&&(mod(VoltageVectorAngleOptimum, 2*pi)>=pi)  % sector 4
        DutyA = (Svpwm_T0/2)/TswSelected;
        DutyB = (Svpwm_T1+Svpwm_T0/2)/TswSelected;
        DutyC = (Svpwm_T1+Svpwm_T2+Svpwm_T0/2)/TswSelected;
%         sectornumber = 4;
        return;
    end
    if (mod(VoltageVectorAngleOptimum, 2*pi)<=5*pi/3)&&(mod(VoltageVectorAngleOptimum, 2*pi)>=4*pi/3)  % sector 5
        DutyA = (Svpwm_T2+Svpwm_T0/2)/TswSelected;
        DutyB = (Svpwm_T0/2)/TswSelected;
        DutyC = (Svpwm_T1+Svpwm_T2+Svpwm_T0/2)/TswSelected;
%         sectornumber = 5;
        return;
    end
    if (mod(VoltageVectorAngleOptimum, 2*pi)<=2*pi)&&(mod(VoltageVectorAngleOptimum, 2*pi)>=5*pi/3)  % sector 6
        DutyA = (Svpwm_T1+Svpwm_T2+Svpwm_T0/2)/TswSelected;
        DutyB = (Svpwm_T0/2)/TswSelected;
        DutyC = (Svpwm_T1+Svpwm_T0/2)/TswSelected;
%         sectornumber = 6;
        return;
    end
    
else %switching pulse
    
    FswSelected = FswSelected_prev;
    DutyA = DutyA_prev;
    DutyB = DutyB_prev;
    DutyC = DutyC_prev;
    IqRipplePrediction = IqRipplePrediction_prev;
end

== matlab function mpc_model_with_pos_est/MATLAB Function ==
  data: id input; pos_est output; iq input; id_1_prev input; iq_1_prev input; vd input; vq input; wmech input; thetamech input; fsw input; speed_est output; pos_est_prev input; speed_prev input; id_1 output; iq_1 output; P_1_prev input; P_1 output; clock input
function [pos_est, speed_est,id_1,iq_1,P_1] = fcn(id,iq,id_1_prev,iq_1_prev,vd,vq,wmech, thetamech, fsw, pos_est_prev,speed_prev,P_1_prev, clock)

% P_1_prev = P_1;

Ls = 0.003510000000000;
Rs = 0.321;
PolePairs = 10;
pos_est = 0;
speed_est = 0;
FluxPM = 0.1808;
id_1 = id + (1/fsw)*(vd/Ls-Rs*id/Ls+wmech*iq*PolePairs);
iq_1 = iq + (1/fsw)*(vq/Ls-Rs*iq/Ls-wmech*id*PolePairs-FluxPM*wmech*PolePairs/Ls);
welec = wmech*PolePairs;
wmech_1 = wmech;
welec_1 = wmech*PolePairs;
thetaelec = thetamech*PolePairs;
thataelec_1 = thetaelec + PolePairs*wmech*(1/fsw);
thetamech_1 = thetamech + wmech*(1/fsw);


td = Ls/Rs;
tq = Ls/Rs;
Te = 1/fsw;
F = [(1-Te/td) (Te*wmech*PolePairs) (Te*iq) 0;(-Te*PolePairs*wmech) (1-Te/tq) (Te*(-id-wmech*FluxPM*PolePairs/Ls)) 0;0 0 1 0; 0 0 Te 1];

if(clock==0)
    P_prev = eye(4)*0.1;
else
    P_prev = P_1_prev;
end

Q = eye(4)*10;
R = eye(2)*0.9;
y = [id iq]';

x_meas = [id iq welec thetaelec]';
x_predict = [id_1 iq_1 welec_1 thataelec_1]';
x_error = x_meas-x_predict;
C = [1 0 0 0;0 1 0 0];
P = F*P_prev*F';

K = P*C'*(C*P*C'+R);

x_est = x_predict + K*(y-C*x_predict);

pos_est = x_est(4);
speed_est = x_est(3);

P_1 = [eye(4)-K*C]*P;

== matlab function mpc_model_with_pos_est/abc to dq0 ==
  data: ids output; iqs output; ias input; ibs input; ics input; ref_frame_position input; i0 output
function [ids,iqs,i0 ]  = fcn(ias,ibs,ics,ref_frame_position)





ids = 2/3*(ias*sin(ref_frame_position)+ibs*sin(ref_frame_position-2*pi/3)+ics*sin(ref_frame_position+2*pi/3));
iqs =  2/3*(ias*cos(ref_frame_position)+ibs*cos(ref_frame_position-2*pi/3)+ics*cos(ref_frame_position+2*pi/3));
i0 = 2/3*1/2*(ias+ibs+ics);
% iqs = (vqs-fluxlinkage_qs_derivative-ref_frame_velocity*fluxlinkage_ds)/rs;
% ids = (vds-fluxlinkage_ds_derivative+ref_frame_velocity*fluxlinkage_qs)/rs;

== matlab function mpc_model_with_pos_est/MATLAB Function1 ==
  data: pulse input; inputwave input; outputwave output
function outputwave  = fcn(pulse, inputwave)

persistent state

if isempty(state)
state = 0;
end

if(pulse==1)
    state = state +1;
end

if(mod(state,2)==1)
    outputwave = inputwave;
    return;
end
if(mod(state,2)==0)
    outputwave = 1-inputwave;
    return;
end

outputwave = 5;
